simulink model "SEIR_Model"  (R2022b)
settings: Solver=ode1  StartTime=0.0  StopTime=2000  FixedStep=5  RelTol=1e-1
undefined symbols (not defined in the file): Alpha, Beta, Gamma, Mue, Omega, Sigma
settings Model: Creator=farru  LastModifiedBy=farru

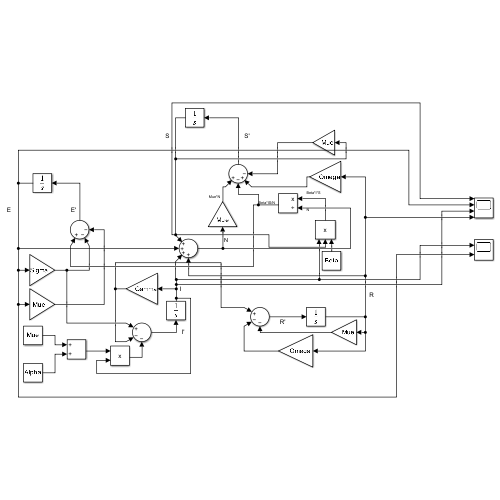
[thumbnail: Simulink's stored preview of the top-level diagram]
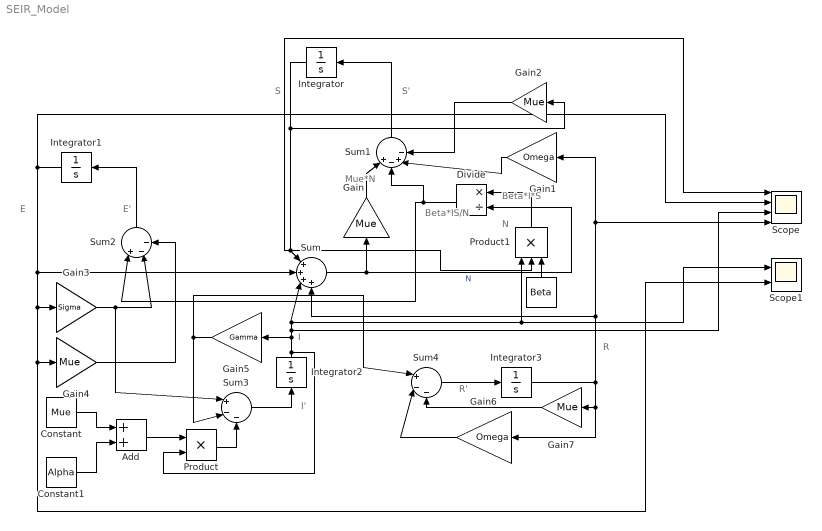
== system SEIR_Model ==
  note: R'
  note: R
  note: I
  note: I'
  note: E
  note: E'
  note: Beta*IS/N
  note: S
  note: S'
  note: Beta*I*S
  note: N
  note: Mue*N
  " " : Constant  Value=Beta
  Add : Sum
  Constant : Constant  Value=Mue
  Constant1 : Constant  Value=Alpha
  Divide : Product  Inputs=*/
  Gain{,2,4,7} (4 alike) : Gain  Gain=Mue
  Gain1 : Gain  Gain=Omega
  Gain3 : Gain  Gain=Sigma
  Gain5 : Gain  Gain=Gamma
  Gain6 : Gain  Gain=Omega
  Integrator : Integrator  InitialCondition=0.999
  Integrator1 : Integrator  InitialCondition=0.001
  Integrator2 : Integrator
  Integrator3 : Integrator
  Product : Product
  Product1 : Product  Inputs=3
  Scope : Scope  NumInputPorts=4
  Scope1 : Scope  NumInputPorts=2
  Sum : Sum  Inputs=|++++
  Sum1 : Sum  Inputs=|+-+-
  Sum2 : Sum  Inputs=|+--
  Sum3 : Sum  Inputs=|+--
  Sum4 : Sum  Inputs=|+--
  wires:
  Sum/1 -> Gain/1, Divide/2  "N"
  Gain/1 -> Sum1/1
  Product1/1 -> Divide/1
  Integrator1/1 -> Scope1/2, Gain4/1, Gain3/1, Sum/2, Scope/2
  Integrator3/1 -> Gain6/1, Gain7/1, Scope/4, Gain1/1, Sum/4
  " "/1 -> Product1/3
  Divide/1 -> Sum2/1, Sum1/2
  Gain1/1 -> Sum1/3
  Gain2/1 -> Sum1/4
  Sum1/1 -> Integrator/1
  Sum2/1 -> Integrator1/1
  Gain3/1 -> Sum3/1, Sum2/2
  Gain4/1 -> Sum2/3
  Sum3/1 -> Integrator2/1
  Gain5/1 -> Sum4/1, Sum3/2
  Constant/1 -> Add/1
  Constant1/1 -> Add/2
  Add/1 -> Product/1
  Product/1 -> Sum3/3
  Integrator2/1 -> Scope/3, Scope1/1, Product1/1, Sum/3, Gain5/1, Product/2
  Sum4/1 -> Integrator3/1
  Gain6/1 -> Sum4/2
  Gain7/1 -> Sum4/3
  Integrator/1 -> Scope/1, Product1/2, Sum/1, Gain2/1
